simulink library "monroe_library"  (R2012b)
settings: Solver=ode45  StartTime=0.0  StopTime=10.0  RelTol=1e-3
values from neighbouring files (symbols this model uses):
  input_bit_width = ', num2str(input_bit_width))    [fft_direct_draw.m]
undefined symbols (not defined in the file or in its folder): gcbh, xlBlockLoadCallback
libraries: xbsIndex_r4 x1880, monroe_library x159, casper_library x13, xps_library x1
(part 8 of 43)

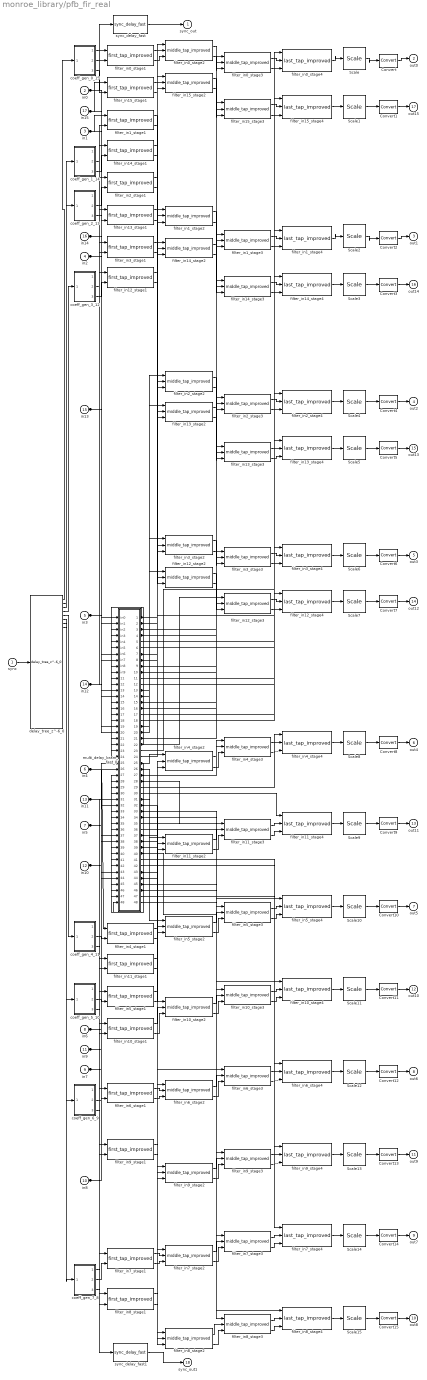
== system monroe_library/pfb_fir_real ==
  sync : Inport
  in0 : Inport  Port=2
  in1 : Inport  Port=3
  in2 : Inport  Port=4
  in3 : Inport  Port=5
  in4 : Inport  Port=6
  in5 : Inport  Port=7
  in6 : Inport  Port=8
  in7 : Inport  Port=9
  in8 : Inport  Port=10
  in9 : Inport  Port=11
  in10 : Inport  Port=12
  in11 : Inport  Port=13
  in12 : Inport  Port=14
  in13 : Inport  Port=15
  in14 : Inport  Port=16
  in15 : Inport  Port=17
  Convert{,1..15} (16 alike) : xbsIndex_r4/Convert  arith_type="Signed  (2's comp)"  n_bits=18  bin_pt=17  quantization=Truncate  overflow=Wrap  en=off  latency=0  dbl_ovrd=off  pipeline=off  block_type=convert
  Scale{,1..15} (16 alike) : xbsIndex_r4/Scale  scale_factor=-1  dbl_ovrd=off  block_type=scale
  coeff_gen_0_15 : Subsystem
  coeff_gen_1_14 : Subsystem
  coeff_gen_2_13 : Subsystem
  coeff_gen_3_12 : Subsystem
  coeff_gen_4_11 : Subsystem
  coeff_gen_5_10 : Subsystem
  coeff_gen_6_9 : Subsystem
  coeff_gen_7_8 : Subsystem
  delay_tree_z^-6_0 : monroe_library/delay_tree_z^-6_0  SystemSampleTime=-1
  filter_in0_stage1 : monroe_library/first_tap_improved  SystemSampleTime=-1  data_bin_pt=17  coeff_bit_width=18
  filter_in0_stage2 : monroe_library/middle_tap_improved  SystemSampleTime=-1  data_bin_pt=17  coeff_bit_width=18  stage_num=2
  filter_in0_stage3 : monroe_library/middle_tap_improved  SystemSampleTime=-1  data_bin_pt=17  coeff_bit_width=18  stage_num=3
  filter_in0_stage4 : monroe_library/last_tap_improved  SystemSampleTime=-1  data_bin_pt=17  coeff_bin_pt=17  stage_num=4
  filter_in10_stage1 : monroe_library/first_tap_improved  SystemSampleTime=-1  data_bin_pt=17  coeff_bit_width=18
  filter_in10_stage2 : monroe_library/middle_tap_improved  SystemSampleTime=-1  data_bin_pt=17  coeff_bit_width=18  stage_num=2
  filter_in10_stage3 : monroe_library/middle_tap_improved  SystemSampleTime=-1  data_bin_pt=17  coeff_bit_width=18  stage_num=3
  filter_in10_stage4 : monroe_library/last_tap_improved  SystemSampleTime=-1  data_bin_pt=17  coeff_bin_pt=17  stage_num=4
  filter_in11_stage1 : monroe_library/first_tap_improved  SystemSampleTime=-1  data_bin_pt=17  coeff_bit_width=18
  filter_in11_stage2 : monroe_library/middle_tap_improved  SystemSampleTime=-1  data_bin_pt=17  coeff_bit_width=18  stage_num=2
  filter_in11_stage3 : monroe_library/middle_tap_improved  SystemSampleTime=-1  data_bin_pt=17  coeff_bit_width=18  stage_num=3
  filter_in11_stage4 : monroe_library/last_tap_improved  SystemSampleTime=-1  data_bin_pt=17  coeff_bin_pt=17  stage_num=4
  filter_in12_stage1 : monroe_library/first_tap_improved  SystemSampleTime=-1  data_bin_pt=17  coeff_bit_width=18
  filter_in12_stage2 : monroe_library/middle_tap_improved  SystemSampleTime=-1  data_bin_pt=17  coeff_bit_width=18  stage_num=2
  filter_in12_stage3 : monroe_library/middle_tap_improved  SystemSampleTime=-1  data_bin_pt=17  coeff_bit_width=18  stage_num=3
  filter_in12_stage4 : monroe_library/last_tap_improved  SystemSampleTime=-1  data_bin_pt=17  coeff_bin_pt=17  stage_num=4
  filter_in13_stage1 : monroe_library/first_tap_improved  SystemSampleTime=-1  data_bin_pt=17  coeff_bit_width=18
  filter_in13_stage2 : monroe_library/middle_tap_improved  SystemSampleTime=-1  data_bin_pt=17  coeff_bit_width=18  stage_num=2
  filter_in13_stage3 : monroe_library/middle_tap_improved  SystemSampleTime=-1  data_bin_pt=17  coeff_bit_width=18  stage_num=3
  filter_in13_stage4 : monroe_library/last_tap_improved  SystemSampleTime=-1  data_bin_pt=17  coeff_bin_pt=17  stage_num=4
  filter_in14_stage1 : monroe_library/first_tap_improved  SystemSampleTime=-1  data_bin_pt=17  coeff_bit_width=18
  filter_in14_stage2 : monroe_library/middle_tap_improved  SystemSampleTime=-1  data_bin_pt=17  coeff_bit_width=18  stage_num=2
  filter_in14_stage3 : monroe_library/middle_tap_improved  SystemSampleTime=-1  data_bin_pt=17  coeff_bit_width=18  stage_num=3
  filter_in14_stage4 : monroe_library/last_tap_improved  SystemSampleTime=-1  data_bin_pt=17  coeff_bin_pt=17  stage_num=4
  filter_in15_stage1 : monroe_library/first_tap_improved  SystemSampleTime=-1  data_bin_pt=17  coeff_bit_width=18
  filter_in15_stage2 : monroe_library/middle_tap_improved  SystemSampleTime=-1  data_bin_pt=17  coeff_bit_width=18  stage_num=2
  filter_in15_stage3 : monroe_library/middle_tap_improved  SystemSampleTime=-1  data_bin_pt=17  coeff_bit_width=18  stage_num=3
  filter_in15_stage4 : monroe_library/last_tap_improved  SystemSampleTime=-1  data_bin_pt=17  coeff_bin_pt=17  stage_num=4
  filter_in1_stage1 : monroe_library/first_tap_improved  SystemSampleTime=-1  data_bin_pt=17  coeff_bit_width=18
  filter_in1_stage2 : monroe_library/middle_tap_improved  SystemSampleTime=-1  data_bin_pt=17  coeff_bit_width=18  stage_num=2
  filter_in1_stage3 : monroe_library/middle_tap_improved  SystemSampleTime=-1  data_bin_pt=17  coeff_bit_width=18  stage_num=3
  filter_in1_stage4 : monroe_library/last_tap_improved  SystemSampleTime=-1  data_bin_pt=17  coeff_bin_pt=17  stage_num=4
  filter_in2_stage1 : monroe_library/first_tap_improved  SystemSampleTime=-1  data_bin_pt=17  coeff_bit_width=18
  filter_in2_stage2 : monroe_library/middle_tap_improved  SystemSampleTime=-1  data_bin_pt=17  coeff_bit_width=18  stage_num=2
  filter_in2_stage3 : monroe_library/middle_tap_improved  SystemSampleTime=-1  data_bin_pt=17  coeff_bit_width=18  stage_num=3
  filter_in2_stage4 : monroe_library/last_tap_improved  SystemSampleTime=-1  data_bin_pt=17  coeff_bin_pt=17  stage_num=4
  filter_in3_stage1 : monroe_library/first_tap_improved  SystemSampleTime=-1  data_bin_pt=17  coeff_bit_width=18
  filter_in3_stage2 : monroe_library/middle_tap_improved  SystemSampleTime=-1  data_bin_pt=17  coeff_bit_width=18  stage_num=2
  filter_in3_stage3 : monroe_library/middle_tap_improved  SystemSampleTime=-1  data_bin_pt=17  coeff_bit_width=18  stage_num=3
  filter_in3_stage4 : monroe_library/last_tap_improved  SystemSampleTime=-1  data_bin_pt=17  coeff_bin_pt=17  stage_num=4
  filter_in4_stage1 : monroe_library/first_tap_improved  SystemSampleTime=-1  data_bin_pt=17  coeff_bit_width=18
  filter_in4_stage2 : monroe_library/middle_tap_improved  SystemSampleTime=-1  data_bin_pt=17  coeff_bit_width=18  stage_num=2
  filter_in4_stage3 : monroe_library/middle_tap_improved  SystemSampleTime=-1  data_bin_pt=17  coeff_bit_width=18  stage_num=3
  filter_in4_stage4 : monroe_library/last_tap_improved  SystemSampleTime=-1  data_bin_pt=17  coeff_bin_pt=17  stage_num=4
  filter_in5_stage1 : monroe_library/first_tap_improved  SystemSampleTime=-1  data_bin_pt=17  coeff_bit_width=18
  filter_in5_stage2 : monroe_library/middle_tap_improved  SystemSampleTime=-1  data_bin_pt=17  coeff_bit_width=18  stage_num=2
  filter_in5_stage3 : monroe_library/middle_tap_improved  SystemSampleTime=-1  data_bin_pt=17  coeff_bit_width=18  stage_num=3
  filter_in5_stage4 : monroe_library/last_tap_improved  SystemSampleTime=-1  data_bin_pt=17  coeff_bin_pt=17  stage_num=4
  filter_in6_stage1 : monroe_library/first_tap_improved  SystemSampleTime=-1  data_bin_pt=17  coeff_bit_width=18
  filter_in6_stage2 : monroe_library/middle_tap_improved  SystemSampleTime=-1  data_bin_pt=17  coeff_bit_width=18  stage_num=2
  filter_in6_stage3 : monroe_library/middle_tap_improved  SystemSampleTime=-1  data_bin_pt=17  coeff_bit_width=18  stage_num=3
  filter_in6_stage4 : monroe_library/last_tap_improved  SystemSampleTime=-1  data_bin_pt=17  coeff_bin_pt=17  stage_num=4
  filter_in7_stage1 : monroe_library/first_tap_improved  SystemSampleTime=-1  data_bin_pt=17  coeff_bit_width=18
  filter_in7_stage2 : monroe_library/middle_tap_improved  SystemSampleTime=-1  data_bin_pt=17  coeff_bit_width=18  stage_num=2
  filter_in7_stage3 : monroe_library/middle_tap_improved  SystemSampleTime=-1  data_bin_pt=17  coeff_bit_width=18  stage_num=3
  filter_in7_stage4 : monroe_library/last_tap_improved  SystemSampleTime=-1  data_bin_pt=17  coeff_bin_pt=17  stage_num=4
  filter_in8_stage1 : monroe_library/first_tap_improved  SystemSampleTime=-1  data_bin_pt=17  coeff_bit_width=18
  filter_in8_stage2 : monroe_library/middle_tap_improved  SystemSampleTime=-1  data_bin_pt=17  coeff_bit_width=18  stage_num=2
  filter_in8_stage3 : monroe_library/middle_tap_improved  SystemSampleTime=-1  data_bin_pt=17  coeff_bit_width=18  stage_num=3
  filter_in8_stage4 : monroe_library/last_tap_improved  SystemSampleTime=-1  data_bin_pt=17  coeff_bin_pt=17  stage_num=4
  filter_in9_stage1 : monroe_library/first_tap_improved  SystemSampleTime=-1  data_bin_pt=17  coeff_bit_width=18
  filter_in9_stage2 : monroe_library/middle_tap_improved  SystemSampleTime=-1  data_bin_pt=17  coeff_bit_width=18  stage_num=2
  filter_in9_stage3 : monroe_library/middle_tap_improved  SystemSampleTime=-1  data_bin_pt=17  coeff_bit_width=18  stage_num=3
  filter_in9_stage4 : monroe_library/last_tap_improved  SystemSampleTime=-1  data_bin_pt=17  coeff_bin_pt=17  stage_num=4
  multi_delay_bram_fast_0 : Subsystem
  sync_delay_fast : monroe_library/sync_delay_fast  SystemSampleTime=-1  delay_len=4102
  sync_delay_fast1 : monroe_library/sync_delay_fast  SystemSampleTime=-1  delay_len=4102
  sync_out : Outport
  out0 : Outport  Port=2
  out1 : Outport  Port=3
  out2 : Outport  Port=4
  out3 : Outport  Port=5
  out4 : Outport  Port=6
  out5 : Outport  Port=7
  out6 : Outport  Port=8
  out7 : Outport  Port=9
  out8 : Outport  Port=10
  out9 : Outport  Port=11
  out10 : Outport  Port=12
  out11 : Outport  Port=13
  out12 : Outport  Port=14
  out13 : Outport  Port=15
  out14 : Outport  Port=16
  out15 : Outport  Port=17
  sync_out1 : Outport  Port=18
  wires:
  in0/1 -> multi_delay_bram_fast_0/1(in0), filter_in0_stage1/1
  in15/1 -> multi_delay_bram_fast_0/2(in1), filter_in15_stage1/1
  in1/1 -> filter_in1_stage1/1, multi_delay_bram_fast_0/7(in6)
  in14/1 -> filter_in14_stage1/1, multi_delay_bram_fast_0/8(in7)
  in2/1 -> filter_in2_stage1/1, multi_delay_bram_fast_0/13(in12)
  in13/1 -> filter_in13_stage1/1, multi_delay_bram_fast_0/14(in13)
  in3/1 -> filter_in3_stage1/1, multi_delay_bram_fast_0/19(in18)
  in12/1 -> filter_in12_stage1/1, multi_delay_bram_fast_0/20(in19)
  in4/1 -> filter_in4_stage1/1, multi_delay_bram_fast_0/25(in24)
  in11/1 -> filter_in11_stage1/1, multi_delay_bram_fast_0/26(in25)
  in5/1 -> filter_in5_stage1/1, multi_delay_bram_fast_0/31(in30)
  in10/1 -> filter_in10_stage1/1, multi_delay_bram_fast_0/32(in31)
  in6/1 -> filter_in6_stage1/1, multi_delay_bram_fast_0/37(in36)
  in9/1 -> filter_in9_stage1/1, multi_delay_bram_fast_0/38(in37)
  in7/1 -> filter_in7_stage1/1, multi_delay_bram_fast_0/43(in42)
  in8/1 -> filter_in8_stage1/1, multi_delay_bram_fast_0/44(in43)
  multi_delay_bram_fast_0/1(out0) -> filter_in0_stage2/1, multi_delay_bram_fast_0/3(in2)
  multi_delay_bram_fast_0/2(out1) -> filter_in15_stage2/1, multi_delay_bram_fast_0/4(in3)
  multi_delay_bram_fast_0/3(out2) -> filter_in0_stage3/1, multi_delay_bram_fast_0/5(in4)
  multi_delay_bram_fast_0/4(out3) -> filter_in15_stage3/1, multi_delay_bram_fast_0/6(in5)
  multi_delay_bram_fast_0/7(out6) -> filter_in1_stage2/1, multi_delay_bram_fast_0/9(in8)
  multi_delay_bram_fast_0/8(out7) -> filter_in14_stage2/1, multi_delay_bram_fast_0/10(in9)
  multi_delay_bram_fast_0/9(out8) -> filter_in1_stage3/1, multi_delay_bram_fast_0/11(in10)
  multi_delay_bram_fast_0/10(out9) -> filter_in14_stage3/1, multi_delay_bram_fast_0/12(in11)
  multi_delay_bram_fast_0/13(out12) -> filter_in2_stage2/1, multi_delay_bram_fast_0/15(in14)
  multi_delay_bram_fast_0/14(out13) -> filter_in13_stage2/1, multi_delay_bram_fast_0/16(in15)
  multi_delay_bram_fast_0/15(out14) -> filter_in2_stage3/1, multi_delay_bram_fast_0/17(in16)
  multi_delay_bram_fast_0/16(out15) -> filter_in13_stage3/1, multi_delay_bram_fast_0/18(in17)
  multi_delay_bram_fast_0/19(out18) -> filter_in3_stage2/1, multi_delay_bram_fast_0/21(in20)
  multi_delay_bram_fast_0/20(out19) -> filter_in12_stage2/1, multi_delay_bram_fast_0/22(in21)
  multi_delay_bram_fast_0/21(out20) -> filter_in3_stage3/1, multi_delay_bram_fast_0/23(in22)
  multi_delay_bram_fast_0/22(out21) -> filter_in12_stage3/1, multi_delay_bram_fast_0/24(in23)
  multi_delay_bram_fast_0/25(out24) -> filter_in4_stage2/1, multi_delay_bram_fast_0/27(in26)
  multi_delay_bram_fast_0/26(out25) -> filter_in11_stage2/1, multi_delay_bram_fast_0/28(in27)
  multi_delay_bram_fast_0/27(out26) -> filter_in4_stage3/1, multi_delay_bram_fast_0/29(in28)
  multi_delay_bram_fast_0/28(out27) -> filter_in11_stage3/1, multi_delay_bram_fast_0/30(in29)
  multi_delay_bram_fast_0/31(out30) -> filter_in5_stage2/1, multi_delay_bram_fast_0/33(in32)
  multi_delay_bram_fast_0/32(out31) -> filter_in10_stage2/1, multi_delay_bram_fast_0/34(in33)
  multi_delay_bram_fast_0/33(out32) -> filter_in5_stage3/1, multi_delay_bram_fast_0/35(in34)
  multi_delay_bram_fast_0/34(out33) -> filter_in10_stage3/1, multi_delay_bram_fast_0/36(in35)
  multi_delay_bram_fast_0/37(out36) -> filter_in6_stage2/1, multi_delay_bram_fast_0/39(in38)
  multi_delay_bram_fast_0/38(out37) -> filter_in9_stage2/1, multi_delay_bram_fast_0/40(in39)
  multi_delay_bram_fast_0/39(out38) -> filter_in6_stage3/1, multi_delay_bram_fast_0/41(in40)
  multi_delay_bram_fast_0/40(out39) -> filter_in9_stage3/1, multi_delay_bram_fast_0/42(in41)
  multi_delay_bram_fast_0/43(out42) -> filter_in7_stage2/1, multi_delay_bram_fast_0/45(in44)
  multi_delay_bram_fast_0/44(out43) -> filter_in8_stage2/1, multi_delay_bram_fast_0/46(in45)
  multi_delay_bram_fast_0/45(out44) -> filter_in7_stage3/1, multi_delay_bram_fast_0/47(in46)
  multi_delay_bram_fast_0/46(out45) -> filter_in8_stage3/1, multi_delay_bram_fast_0/48(in47)
  sync_delay_fast1/1 -> sync_out1/1
  coeff_gen_7_8/1(sync_out) -> sync_delay_fast1/1
  sync_delay_fast/1 -> sync_out/1
  coeff_gen_0_15/1(sync_out) -> sync_delay_fast/1
  Convert15/1 -> out8/1
  Scale15/1 -> Convert15/1
  Convert14/1 -> out7/1
  Scale14/1 -> Convert14/1
  filter_in8_stage4/1 -> Scale15/1
  filter_in7_stage4/1 -> Scale14/1
  filter_in8_stage3/2 -> filter_in8_stage4/3
  filter_in8_stage3/1 -> filter_in8_stage4/2
  multi_delay_bram_fast_0/48(out47) -> filter_in8_stage4/1
  filter_in7_stage3/2 -> filter_in7_stage4/3
  filter_in7_stage3/1 -> filter_in7_stage4/2
  multi_delay_bram_fast_0/47(out46) -> filter_in7_stage4/1
  filter_in8_stage2/2 -> filter_in8_stage3/3
  filter_in8_stage2/1 -> filter_in8_stage3/2
  filter_in7_stage2/2 -> filter_in7_stage3/3
  filter_in7_stage2/1 -> filter_in7_stage3/2
  filter_in8_stage1/2 -> filter_in8_stage2/3
  filter_in8_stage1/1 -> filter_in8_stage2/2
  filter_in7_stage1/2 -> filter_in7_stage2/3
  filter_in7_stage1/1 -> filter_in7_stage2/2
  coeff_gen_7_8/3(coeff_rev) -> filter_in8_stage1/2
  coeff_gen_7_8/2(coeff) -> filter_in7_stage1/2
  delay_tree_z^-6_0/8 -> coeff_gen_7_8/1(sync)
  Convert13/1 -> out9/1
  Scale13/1 -> Convert13/1
  Convert12/1 -> out6/1
  Scale12/1 -> Convert12/1
  filter_in9_stage4/1 -> Scale13/1
  filter_in6_stage4/1 -> Scale12/1
  filter_in9_stage3/2 -> filter_in9_stage4/3
  filter_in9_stage3/1 -> filter_in9_stage4/2
  multi_delay_bram_fast_0/42(out41) -> filter_in9_stage4/1
  filter_in6_stage3/2 -> filter_in6_stage4/3
  filter_in6_stage3/1 -> filter_in6_stage4/2
  multi_delay_bram_fast_0/41(out40) -> filter_in6_stage4/1
  filter_in9_stage2/2 -> filter_in9_stage3/3
  filter_in9_stage2/1 -> filter_in9_stage3/2
  filter_in6_stage2/2 -> filter_in6_stage3/3
  filter_in6_stage2/1 -> filter_in6_stage3/2
  filter_in9_stage1/2 -> filter_in9_stage2/3
  filter_in9_stage1/1 -> filter_in9_stage2/2
  filter_in6_stage1/2 -> filter_in6_stage2/3
  filter_in6_stage1/1 -> filter_in6_stage2/2
  coeff_gen_6_9/3(coeff_rev) -> filter_in9_stage1/2
  coeff_gen_6_9/2(coeff) -> filter_in6_stage1/2
  delay_tree_z^-6_0/7 -> coeff_gen_6_9/1(sync)
  Convert11/1 -> out10/1
  Scale11/1 -> Convert11/1
  Convert10/1 -> out5/1
  Scale10/1 -> Convert10/1
  filter_in10_stage4/1 -> Scale11/1
  filter_in5_stage4/1 -> Scale10/1
  filter_in10_stage3/2 -> filter_in10_stage4/3
  filter_in10_stage3/1 -> filter_in10_stage4/2
  multi_delay_bram_fast_0/36(out35) -> filter_in10_stage4/1
  filter_in5_stage3/2 -> filter_in5_stage4/3
  filter_in5_stage3/1 -> filter_in5_stage4/2
  multi_delay_bram_fast_0/35(out34) -> filter_in5_stage4/1
  filter_in10_stage2/2 -> filter_in10_stage3/3
  filter_in10_stage2/1 -> filter_in10_stage3/2
  filter_in5_stage2/2 -> filter_in5_stage3/3
  filter_in5_stage2/1 -> filter_in5_stage3/2
  filter_in10_stage1/2 -> filter_in10_stage2/3
  filter_in10_stage1/1 -> filter_in10_stage2/2
  filter_in5_stage1/2 -> filter_in5_stage2/3
  filter_in5_stage1/1 -> filter_in5_stage2/2
  coeff_gen_5_10/3(coeff_rev) -> filter_in10_stage1/2
  coeff_gen_5_10/2(coeff) -> filter_in5_stage1/2
  delay_tree_z^-6_0/6 -> coeff_gen_5_10/1(sync)
  Convert9/1 -> out11/1
  Scale9/1 -> Convert9/1
  Convert8/1 -> out4/1
  Scale8/1 -> Convert8/1
  filter_in11_stage4/1 -> Scale9/1
  filter_in4_stage4/1 -> Scale8/1
  filter_in11_stage3/2 -> filter_in11_stage4/3
  filter_in11_stage3/1 -> filter_in11_stage4/2
  multi_delay_bram_fast_0/30(out29) -> filter_in11_stage4/1
  filter_in4_stage3/2 -> filter_in4_stage4/3
  filter_in4_stage3/1 -> filter_in4_stage4/2
  multi_delay_bram_fast_0/29(out28) -> filter_in4_stage4/1
  filter_in11_stage2/2 -> filter_in11_stage3/3
  filter_in11_stage2/1 -> filter_in11_stage3/2
  filter_in4_stage2/2 -> filter_in4_stage3/3
  filter_in4_stage2/1 -> filter_in4_stage3/2
  filter_in11_stage1/2 -> filter_in11_stage2/3
  filter_in11_stage1/1 -> filter_in11_stage2/2
  filter_in4_stage1/2 -> filter_in4_stage2/3
  filter_in4_stage1/1 -> filter_in4_stage2/2
  coeff_gen_4_11/3(coeff_rev) -> filter_in11_stage1/2
  coeff_gen_4_11/2(coeff) -> filter_in4_stage1/2
  delay_tree_z^-6_0/5 -> coeff_gen_4_11/1(sync)
  Convert7/1 -> out12/1
  Scale7/1 -> Convert7/1
  Convert6/1 -> out3/1
  Scale6/1 -> Convert6/1
  filter_in12_stage4/1 -> Scale7/1
  filter_in3_stage4/1 -> Scale6/1
  filter_in12_stage3/2 -> filter_in12_stage4/3
  filter_in12_stage3/1 -> filter_in12_stage4/2
  multi_delay_bram_fast_0/24(out23) -> filter_in12_stage4/1
  filter_in3_stage3/2 -> filter_in3_stage4/3
  filter_in3_stage3/1 -> filter_in3_stage4/2
  multi_delay_bram_fast_0/23(out22) -> filter_in3_stage4/1
  filter_in12_stage2/2 -> filter_in12_stage3/3
  filter_in12_stage2/1 -> filter_in12_stage3/2
  filter_in3_stage2/2 -> filter_in3_stage3/3
  filter_in3_stage2/1 -> filter_in3_stage3/2
  filter_in12_stage1/2 -> filter_in12_stage2/3
  filter_in12_stage1/1 -> filter_in12_stage2/2
  filter_in3_stage1/2 -> filter_in3_stage2/3
  filter_in3_stage1/1 -> filter_in3_stage2/2
  coeff_gen_3_12/3(coeff_rev) -> filter_in12_stage1/2
  coeff_gen_3_12/2(coeff) -> filter_in3_stage1/2
  delay_tree_z^-6_0/4 -> coeff_gen_3_12/1(sync)
  Convert5/1 -> out13/1
  Scale5/1 -> Convert5/1
  Convert4/1 -> out2/1
  Scale4/1 -> Convert4/1
  filter_in13_stage4/1 -> Scale5/1
  filter_in2_stage4/1 -> Scale4/1
  filter_in13_stage3/2 -> filter_in13_stage4/3
  filter_in13_stage3/1 -> filter_in13_stage4/2
  multi_delay_bram_fast_0/18(out17) -> filter_in13_stage4/1
  filter_in2_stage3/2 -> filter_in2_stage4/3
  filter_in2_stage3/1 -> filter_in2_stage4/2
  multi_delay_bram_fast_0/17(out16) -> filter_in2_stage4/1
  filter_in13_stage2/2 -> filter_in13_stage3/3
  filter_in13_stage2/1 -> filter_in13_stage3/2
  filter_in2_stage2/2 -> filter_in2_stage3/3
  filter_in2_stage2/1 -> filter_in2_stage3/2
  filter_in13_stage1/2 -> filter_in13_stage2/3
  filter_in13_stage1/1 -> filter_in13_stage2/2
  filter_in2_stage1/2 -> filter_in2_stage2/3
  filter_in2_stage1/1 -> filter_in2_stage2/2
  coeff_gen_2_13/3(coeff_rev) -> filter_in13_stage1/2
  coeff_gen_2_13/2(coeff) -> filter_in2_stage1/2
  delay_tree_z^-6_0/3 -> coeff_gen_2_13/1(sync)
  Convert3/1 -> out14/1
  Scale3/1 -> Convert3/1
  Convert2/1 -> out1/1
  Scale2/1 -> Convert2/1
  filter_in14_stage4/1 -> Scale3/1
  filter_in1_stage4/1 -> Scale2/1
  filter_in14_stage3/2 -> filter_in14_stage4/3
  filter_in14_stage3/1 -> filter_in14_stage4/2
  multi_delay_bram_fast_0/12(out11) -> filter_in14_stage4/1
  filter_in1_stage3/2 -> filter_in1_stage4/3
  filter_in1_stage3/1 -> filter_in1_stage4/2
  multi_delay_bram_fast_0/11(out10) -> filter_in1_stage4/1
  filter_in14_stage2/2 -> filter_in14_stage3/3
  filter_in14_stage2/1 -> filter_in14_stage3/2
  filter_in1_stage2/2 -> filter_in1_stage3/3
  filter_in1_stage2/1 -> filter_in1_stage3/2
  filter_in14_stage1/2 -> filter_in14_stage2/3
  filter_in14_stage1/1 -> filter_in14_stage2/2
  filter_in1_stage1/2 -> filter_in1_stage2/3
  filter_in1_stage1/1 -> filter_in1_stage2/2
  coeff_gen_1_14/3(coeff_rev) -> filter_in14_stage1/2
  coeff_gen_1_14/2(coeff) -> filter_in1_stage1/2
  delay_tree_z^-6_0/2 -> coeff_gen_1_14/1(sync)
  Convert1/1 -> out15/1
  Scale1/1 -> Convert1/1
  Convert/1 -> out0/1
  Scale/1 -> Convert/1
  filter_in15_stage4/1 -> Scale1/1
  filter_in0_stage4/1 -> Scale/1
  filter_in15_stage3/2 -> filter_in15_stage4/3
  filter_in15_stage3/1 -> filter_in15_stage4/2
  multi_delay_bram_fast_0/6(out5) -> filter_in15_stage4/1
  filter_in0_stage3/2 -> filter_in0_stage4/3
  filter_in0_stage3/1 -> filter_in0_stage4/2
  multi_delay_bram_fast_0/5(out4) -> filter_in0_stage4/1
  filter_in15_stage2/2 -> filter_in15_stage3/3
  filter_in15_stage2/1 -> filter_in15_stage3/2
  filter_in0_stage2/2 -> filter_in0_stage3/3
  filter_in0_stage2/1 -> filter_in0_stage3/2
  filter_in15_stage1/2 -> filter_in15_stage2/3
  filter_in15_stage1/1 -> filter_in15_stage2/2
  filter_in0_stage1/2 -> filter_in0_stage2/3
  filter_in0_stage1/1 -> filter_in0_stage2/2
  coeff_gen_0_15/3(coeff_rev) -> filter_in15_stage1/2
  coeff_gen_0_15/2(coeff) -> filter_in0_stage1/2
  delay_tree_z^-6_0/1 -> coeff_gen_0_15/1(sync)
  sync/1 -> delay_tree_z^-6_0/1

== system monroe_library/pow_dsp48e ==
  a : Inport
  Convert1 : xbsIndex_r4/Convert  arith_type="Signed  (2's comp)"  n_bits=18  bin_pt=bit_width-1  quantization=Truncate  overflow=Wrap  en=off  latency=0  dbl_ovrd=off  pipeline=off  block_type=convert
      settings: block_version=11.3
  Convert2 : xbsIndex_r4/Convert  arith_type="Signed  (2's comp)"  n_bits=18  bin_pt=bit_width-1  quantization=Truncate  overflow=Wrap  en=off  latency=0  dbl_ovrd=off  pipeline=off  block_type=convert
      settings: block_version=11.3
  Convert3 : xbsIndex_r4/Convert  arith_type="Signed  (2's comp)"  n_bits=30  bin_pt=bit_width-1  quantization=Truncate  overflow=Wrap  en=off  latency=0  dbl_ovrd=off  pipeline=off  block_type=convert
      settings: block_version=11.3
  Convert4 : xbsIndex_r4/Convert  arith_type="Signed  (2's comp)"  n_bits=30  bin_pt=bit_width-1  quantization=Truncate  overflow=Wrap  en=off  latency=0  dbl_ovrd=off  pipeline=off  block_type=convert
      settings: block_version=11.3
  Convert5 : xbsIndex_r4/Convert  arith_type="Signed  (2's comp)"  n_bits=bit_width*2  bin_pt=(bit_width-1)*2  quantization=Truncate  overflow=Wrap  en=off  latency=0  dbl_ovrd=off  pipeline=off  block_type=convert
      settings: block_version=11.3
  Reinterpret{1..4} (4 alike) : xbsIndex_r4/Reinterpret  force_arith_type=on  arith_type="Signed  (2's comp)"  force_bin_pt=on  bin_pt=0  block_type=reinterpret
      settings: infoedit="Changes signal type without altering the binary representation.   You can changed the signal between signed and unsigned, and relocate the binary point.<br><br>Hardware notes: In hardware this block costs nothing.<br><br>Example:  Suppose the input is 6 bits wide, signed, with 2 fractional bits, and the output is forced to unsigned with 0 fractional bits.  Then an input of -2.0 (1110.00 in binary 2's complement) becomes an output of 56 (111000 in binary)."  block_version=11.3
  Reinterpret5 : xbsIndex_r4/Reinterpret  force_arith_type=on  arith_type="Signed  (2's comp)"  force_bin_pt=on  bin_pt=(bit_width - 1)*2  block_type=reinterpret
      settings: infoedit="Changes signal type without altering the binary representation.   You can changed the signal between signed and unsigned, and relocate the binary point.<br><br>Hardware notes: In hardware this block costs nothing.<br><br>Example:  Suppose the input is 6 bits wide, signed, with 2 fractional bits, and the output is forced to unsigned with 0 fractional bits.  Then an input of -2.0 (1110.00 in binary 2's complement) becomes an output of 56 (111000 in binary)."  block_version=11.3
  Terminator : Terminator
  Terminator1 : Terminator
  alucode : xbsIndex_r4/Constant  arith_type=Unsigned  const=0  n_bits=4  bin_pt=0  explicit_period=on  period=1  equ=P=C  opselect=C  inp2=PCIN>>17  opr=+  inp1=P  carry=CIN  dbl_ovrd=off  block_type=constant
  alucode1 : xbsIndex_r4/Constant  arith_type=Unsigned  const=0  n_bits=4  bin_pt=0  explicit_period=on  period=1  equ=P=C  opselect=C  inp2=PCIN>>17  opr=+  inp1=P  carry=CIN  dbl_ovrd=off  block_type=constant
  c_to_ri : casper_library/Misc/c_to_ri  SystemSampleTime=-1  n_bits=bit_width  bin_pt=bit_width-1
      settings: AttributesFormatString=8_7 r/i
  carryin : xbsIndex_r4/Constant  arith_type=Unsigned  const=0  n_bits=1  bin_pt=0  explicit_period=on  period=1  equ=P=C  opselect=C  inp2=PCIN>>17  opr=+  inp1=P  carry=CIN  dbl_ovrd=off  block_type=constant
  carryin1 : xbsIndex_r4/Constant  arith_type=Unsigned  const=0  n_bits=1  bin_pt=0  explicit_period=on  period=1  equ=P=C  opselect=C  inp2=PCIN>>17  opr=+  inp1=P  carry=CIN  dbl_ovrd=off  block_type=constant
  carryinsel : xbsIndex_r4/Constant  arith_type=Unsigned  const=0  n_bits=3  bin_pt=0  explicit_period=on  period=1  equ=P=C  opselect=C  inp2=PCIN>>17  opr=+  inp1=P  carry=CIN  dbl_ovrd=off  block_type=constant
  carryinsel1 : xbsIndex_r4/Constant  arith_type=Unsigned  const=0  n_bits=3  bin_pt=0  explicit_period=on  period=1  equ=P=C  opselect=C  inp2=PCIN>>17  opr=+  inp1=P  carry=CIN  dbl_ovrd=off  block_type=constant
  imag_sq : xbsIndex_r4/DSP48E  use_a=Direct from A Port  use_b=Direct from B Port  reset_preg=off  pattern_from_creg=off  pattern='000000000000'  mask_from_creg=off  pattern_mask='3FFFFFFFFFFF'  sel_rounding_mask=Select mask  use_op=off  use_creg=off  rst_all=off  en_all=off  use_pcin=off  use_carrycascin=off  use_multsignin=off  use_carryout=off  use_patterndetect=off  use_patternbdetect=off  use_overflow=off  use_underflow=off  use_acout=off  use_bcout=off  use_pcout=on  use_multsignout=off  use_carrycascout=off  pipeline_a=1  pipeline_b=1  pipeline_acout=1  pipeline_bcout=1  pipeline_c=on  pipeline_p=on  pipeline_mult=on  pipeline_opmode=on  pipeline_alumode=on  pipeline_carryin=on  pipeline_carryinsel=on  rst_a=off  rst_b=off  rst_c=off  rst_mult=off  rst_p=off  rst_carry_in=off  rst_alumode=off  rst_ctrl=off  en_a1=off  en_a2=off  en_b1=off  en_b2=off  en_c=off  en_mult=off  en_p=off  en_carry_in=off  en_alumode=off  en_multcarryin=off  en_ctrl=off  use_synth_model=off  addsub_mode=ONE48  xl_useadderonly=off  block_type=dsp48e
      settings: block_version=10.1.3
  opcode : xbsIndex_r4/Constant  arith_type=Unsigned  const=21  n_bits=7  bin_pt=0  explicit_period=on  period=1  equ=P=C  opselect=C  inp2=PCIN>>17  opr=+  inp1=P  carry=CIN  dbl_ovrd=off  block_type=constant
  opcode1 : xbsIndex_r4/Constant  arith_type=Unsigned  const=5  n_bits=7  bin_pt=0  explicit_period=on  period=1  equ=P=C  opselect=C  inp2=PCIN>>17  opr=+  inp1=P  carry=CIN  dbl_ovrd=off  block_type=constant
  real_sq : xbsIndex_r4/DSP48E  use_a=Direct from A Port  use_b=Direct from B Port  reset_preg=off  pattern_from_creg=off  pattern='000000000000'  mask_from_creg=off  pattern_mask='3FFFFFFFFFFF'  sel_rounding_mask=Select mask  use_op=off  use_creg=off  rst_all=off  en_all=off  use_pcin=on  use_carrycascin=off  use_multsignin=off  use_carryout=off  use_patterndetect=off  use_patternbdetect=off  use_overflow=off  use_underflow=off  use_acout=off  use_bcout=off  use_pcout=on  use_multsignout=off  use_carrycascout=off  pipeline_a=2  pipeline_b=2  pipeline_acout=1  pipeline_bcout=1  pipeline_c=on  pipeline_p=on  pipeline_mult=on  pipeline_opmode=on  pipeline_alumode=on  pipeline_carryin=on  pipeline_carryinsel=on  rst_a=off  rst_b=off  rst_c=off  rst_mult=off  rst_p=off  rst_carry_in=off  rst_alumode=off  rst_ctrl=off  en_a1=off  en_a2=off  en_b1=off  en_b2=off  en_c=off  en_mult=off  en_p=off  en_carry_in=off  en_alumode=off  en_multcarryin=off  en_ctrl=off  use_synth_model=off  addsub_mode=ONE48  xl_useadderonly=off  block_type=dsp48e
      settings: block_version=10.1.3
  pow : Outport
  wires:
  carryinsel1/1 -> imag_sq/6
  carryin1/1 -> imag_sq/5
  alucode1/1 -> imag_sq/4
  opcode1/1 -> imag_sq/3
  imag_sq/2 -> real_sq/3
  opcode/1 -> real_sq/4
  alucode/1 -> real_sq/5
  carryin/1 -> real_sq/6
  carryinsel/1 -> real_sq/7
  imag_sq/1 -> Terminator/1
  real_sq/2 -> Terminator1/1
  real_sq/1 -> Reinterpret5/1
  a/1 -> c_to_ri/1
  c_to_ri/1 -> Convert3/1, Convert2/1
  c_to_ri/2 -> Convert4/1, Convert1/1
  Convert4/1 -> Reinterpret1/1
  Reinterpret1/1 -> imag_sq/1
  Convert1/1 -> Reinterpret2/1
  Reinterpret2/1 -> imag_sq/2
  Convert3/1 -> Reinterpret3/1
  Reinterpret3/1 -> real_sq/1
  Convert2/1 -> Reinterpret4/1
  Reinterpret4/1 -> real_sq/2
  Convert5/1 -> pow/1
  Reinterpret5/1 -> Convert5/1

== system monroe_library/ri_to_c ==
  re : Inport
  im : Inport  Port=2
  concat : xbsIndex_r4/Concat  num_inputs=2  dbl_ovrd=off  block_type=concat
      settings: block_version=9.1.01
  force_im : xbsIndex_r4/Reinterpret  force_arith_type=on  arith_type=Unsigned  force_bin_pt=on  bin_pt=0  block_type=reinterpret
      settings: infoedit="Changes signal type without altering the binary representation.   You can changed the signal between signed and unsigned, and relocate the binary point.<P><P>Hardware notes: In hardware this block costs nothing.<P><P>Example:  Suppose the input is 6 bits wide, signed, with 2 fractional bits, and the output is forced to unsigned with 0 fractional bits.  Then an input of -2.0 (1110.00 in binary 2's complement) becomes an output of 56 (111000 in binary)."  block_version=9.1.01
  force_re : xbsIndex_r4/Reinterpret  force_arith_type=on  arith_type=Unsigned  force_bin_pt=on  bin_pt=0  block_type=reinterpret
      settings: infoedit="Changes signal type without altering the binary representation.   You can changed the signal between signed and unsigned, and relocate the binary point.<P><P>Hardware notes: In hardware this block costs nothing.<P><P>Example:  Suppose the input is 6 bits wide, signed, with 2 fractional bits, and the output is forced to unsigned with 0 fractional bits.  Then an input of -2.0 (1110.00 in binary 2's complement) becomes an output of 56 (111000 in binary)."  block_version=9.1.01
  c : Outport
  wires:
  im/1 -> force_im/1
  concat/1 -> c/1
  re/1 -> force_re/1
  force_im/1 -> concat/2
  force_re/1 -> concat/1

== system monroe_library/sync_delay_fast ==
  in : Inport
  Constant : xbsIndex_r4/Constant  arith_type=Unsigned  const=1  n_bits=ceil(log(delay_len-2)/log(2))  bin_pt=0  explicit_period=on  period=1  equ=P=C  opselect=C  inp2=PCIN>>17  opr=+  inp1=P  carry=CIN  dbl_ovrd=off  block_type=constant
      settings: block_version=9.1.01
  Constant2 : xbsIndex_r4/Constant  arith_type=Unsigned  const=delay_len-3  n_bits=ceil(log(delay_len-2)/log(2))  bin_pt=0  explicit_period=off  period=1  equ=P=C  opselect=C  inp2=PCIN>>17  opr=+  inp1=P  carry=CIN  dbl_ovrd=off  block_type=constant
      settings: block_version=9.1.01
  Counter : xbsIndex_r4/Counter  cnt_type=Free Running  cnt_to=Inf  operation=Down  start_count=0  cnt_by_val=1  arith_type=Unsigned  n_bits=ceil(log(delay_len-2)/log(2))  bin_pt=0  load_pin=on  rst=off  en=on  explicit_period=on  period=1  dbl_ovrd=off  use_behavioral_HDL=on  implementation=Fabric  use_rpm=on  block_type=counter
      settings: xl_area=[0, 0, 0, 0, 0, 0, 0]  block_version=9.1.01
  Delay : xbsIndex_r4/Delay  en=off  latency=2  dbl_ovrd=off  reg_retiming=off  block_type=delay
      settings: block_version=11.4
  Inverter : xbsIndex_r4/Inverter  en=off  latency=0  dbl_ovrd=off  block_type=inv
      settings: block_version=11.4
  Logical : xbsIndex_r4/Logical  logical_function=AND  inputs=2  en=off  latency=1  precision=Full  arith_type=Unsigned  n_bits=16  bin_pt=0  align_bp=on  dbl_ovrd=off  block_type=logical
      settings: block_version=11.4
  Register : xbsIndex_r4/Register  init=0  rst=off  en=on  dbl_ovrd=off  block_type=register
      settings: block_version=11.4
  Register1 : xbsIndex_r4/Register  init=0  rst=off  en=on  dbl_ovrd=off  block_type=register
      settings: block_version=11.4
  Relational : xbsIndex_r4/Relational  mode=a=b  en=off  latency=1  dbl_ovrd=off  block_type=relational
      settings: xl_area=[0, 0, 0, 0, 0, 0, 0]  block_version=9.1.01
  out : Outport
  wires:
  Inverter/1 -> Logical/2
  Delay/1 -> Counter/1
  Logical/1 -> Counter/3
  Register1/1 -> Logical/1
  Register/1 -> Inverter/1
  Relational/1 -> Register/1, Register/2, out/1
  Constant2/1 -> Counter/2
  Constant/1 -> Relational/1
  Counter/1 -> Relational/2
  in/1 -> Delay/1, Register1/1, Register1/2
